simulink model "task9_visu_v23_beide_modelle"  (R2023b)
settings: Solver=VariableStepAuto  StartTime=0.0  StopTime=3  RelTol=1e-3
values from neighbouring files (symbols this model uses):
  tInterval = [0 5]    [task7b.m]    (also in task7b2.m; task8b_setup.m = [0 10]; task9_visu.m = [0 10]; task9b_setup.m = [0 10])
undefined symbols (not defined in the file or in its folder): eul2tform, trvec2tform
libraries: robotcorelib x6, robotmaniplib x4
settings Model: Creator=laith  LastModifiedBy=Nico
settings RTWCC: GPUComputeCapability=5.0

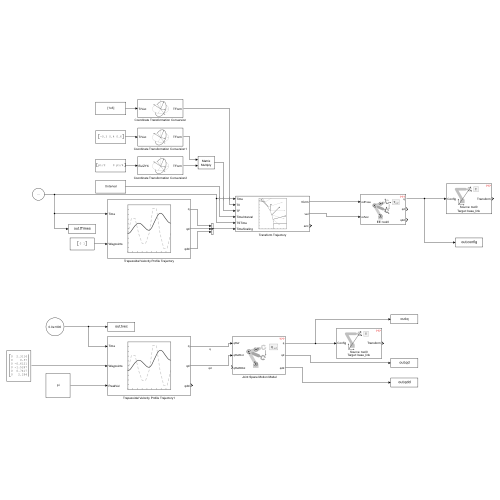
[thumbnail: Simulink's stored preview of the top-level diagram]
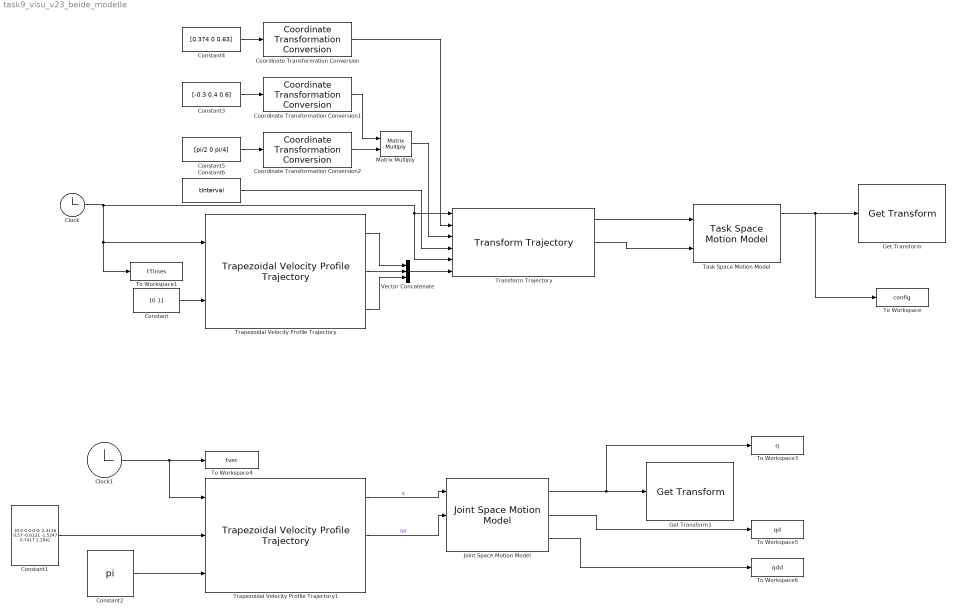
== system task9_visu_v23_beide_modelle ==
  " Joint Space Motion Model" : robotmaniplib/Joint Space Motion Model  RigidBodyTree=robotRBT  MotionType=PD Control  ProportionalGain=200  DerivativeGain=50  ErrorDynamicsSpecification=Damping Ratio / Natural Frequency  DampingRatio=1  NaturalFrequency=10  SettlingTime=0.59  Overshoot=0  ShowExternalForcePort=off  InitConfig=[0 0 0 0 0 0]  InitJointVel=0  SimulateUsing=Interpreted execution
  Clock : Clock
      settings: Decimation=100
  Clock1 : Clock
      settings: Decimation=100
  Constant : Constant  Value=[0 1]  VectorParams1D=off
  Constant1 : Constant  Value="[0 0 0 0 0 0;  2.3116  0.57  -0.6121   -1.5247 0.7417    2.294]'"
  Constant2 : Constant  Value=pi
  Constant3 : Constant  Value=[-0.3 0.4 0.6]
  Constant4 : Constant  Value=[0.374 0 0.63]
  Constant5 : Constant  Value=[pi/2 0 pi/4]
  Constant6 : Constant  Value=tInterval
  Coordinate Transformation Conversion : robotcorelib/Coordinate Transformation Conversion  InputRepresentation=Translation Vector  InputEulerSequence=ZYX  ShowTrVecInputPort=on  OutputRepresentation=Homogeneous Transformation  OutputEulerSequence=ZYX  ShowTrVecOutputPort=on  SimulateUsing=Interpreted execution
  Coordinate Transformation Conversion1 : robotcorelib/Coordinate Transformation Conversion  InputRepresentation=Translation Vector  InputEulerSequence=ZYX  ShowTrVecInputPort=on  OutputRepresentation=Homogeneous Transformation  OutputEulerSequence=ZYX  ShowTrVecOutputPort=off  SimulateUsing=Interpreted execution
  Coordinate Transformation Conversion2 : robotcorelib/Coordinate Transformation Conversion  InputRepresentation=Euler Angles  InputEulerSequence=ZYX  ShowTrVecInputPort=off  OutputRepresentation=Homogeneous Transformation  OutputEulerSequence=ZYX  ShowTrVecOutputPort=on  SimulateUsing=Interpreted execution
  Get Transform : robotmaniplib/Get Transform  RigidBodyTree=robotRBT  SourceBody=tool0  TargetBody=base_link  SimulateUsing=Interpreted execution
  Get Transform1 : robotmaniplib/Get Transform  RigidBodyTree=robotRBT  SourceBody=tool0  TargetBody=base_link  SimulateUsing=Interpreted execution
  Matrix Multiply : Product  Multiplication=Matrix(*)
  Task Space Motion Model : robotmaniplib/Task Space Motion Model  RigidBodyTree=robotRBT  EndEffector=tool0  ProportionalGain=500*eye(6)  DerivativeGain=100*eye(6)  JointDamping=1  ShowExternalForcePort=off  InitConfig=[0 0 0 0 0 0]  InitJointVel=0  SimulateUsing=Interpreted execution
  To Workspace : ToWorkspace  VariableName=config  SampleTime=-1
  To Workspace1 : ToWorkspace  VariableName=tTimes  SampleTime=-1
  To Workspace3 : ToWorkspace  VariableName=q  SampleTime=-1
      settings: Save2DSignal=2-D array (concatenate along first dimension)
  To Workspace4 : ToWorkspace  VariableName=tvec  SampleTime=-1
  To Workspace5 : ToWorkspace  VariableName=qd  SampleTime=-1
      settings: Save2DSignal=2-D array (concatenate along first dimension)
  To Workspace6 : ToWorkspace  VariableName=qdd  SampleTime=-1
      settings: Save2DSignal=2-D array (concatenate along first dimension)
  Transform Trajectory : robotcorelib/Transform Trajectory  WaypointSource=External  T0=trvec2tform( [ 1, 10, -1 ] )  TF=eul2tform( [ 0, pi, pi / 2 ] )  TimeInterval=[ 2, 3 ]  CustomTimeScaling=on  ParameterSource=External  TSTime=2:0.1:3  TimeScaling=[ 0:0.1:1; ones( 1, 11 ); zeros( 1, 11 ) ]  SimulateUsing=Interpreted execution
      settings: LibrarySourceBlock=robotutilslib/Transform Trajectory
  Trapezoidal Velocity Profile Trajectory : robotcorelib/Trapezoidal Velocity Profile Trajectory  WaypointSource=External  Waypoints=[ 0, -0.5, -1; 0, 0.5, 1 ]  NumParams=0  Parameter1=End Time  Parameter2=End Time  ParameterSource=External  PeakVelocity=[ 2; 2 ]  Acceleration=[ 1; 2 ]  EndTime=[ 1; 1 ]  AccelTime=[ 1; 2 ]  SimulateUsing=Code generation
  Trapezoidal Velocity Profile Trajectory1 : robotcorelib/Trapezoidal Velocity Profile Trajectory  WaypointSource=External  Waypoints=[ 0, -0.5, -1; 0, 0.5, 1 ]  NumParams=1  Parameter1=Peak Velocity  Parameter2=Acceleration  ParameterSource=External  PeakVelocity=[ 2; 2 ]  Acceleration=[ 1; 2 ]  EndTime=[ 1; 1 ]  AccelTime=[ 1; 2 ]  SimulateUsing=Interpreted execution
  Vector Concatenate : Concatenate  NumInputs=3  Mode=Multidimensional array
  wires:
  Constant5/1 -> Coordinate Transformation Conversion2/1
  Task Space Motion Model/1 -> To Workspace/1, Get Transform/1
  Transform Trajectory/2 -> Task Space Motion Model/2
  Vector Concatenate/1 -> Transform Trajectory/6
  Constant3/1 -> Coordinate Transformation Conversion1/1
  Coordinate Transformation Conversion/1 -> Transform Trajectory/2
  Trapezoidal Velocity Profile Trajectory/3 -> Vector Concatenate/3
  Trapezoidal Velocity Profile Trajectory/1 -> Vector Concatenate/1
  Constant/1 -> Trapezoidal Velocity Profile Trajectory/2
  Coordinate Transformation Conversion1/1 -> Matrix Multiply/1
  Coordinate Transformation Conversion2/1 -> Matrix Multiply/2
  Matrix Multiply/1 -> Transform Trajectory/3
  Constant4/1 -> Coordinate Transformation Conversion/1
  Trapezoidal Velocity Profile Trajectory/2 -> Vector Concatenate/2
  Clock/1 -> To Workspace1/1, Trapezoidal Velocity Profile Trajectory/1, Transform Trajectory/1, Transform Trajectory/5
  Constant6/1 -> Transform Trajectory/4
  Transform Trajectory/1 -> Task Space Motion Model/1
  Trapezoidal Velocity Profile Trajectory1/2 -> " Joint Space Motion Model"/2  "qd"
  " Joint Space Motion Model"/1 -> To Workspace3/1, Get Transform1/1
  Clock1/1 -> Trapezoidal Velocity Profile Trajectory1/1, To Workspace4/1
  Constant1/1 -> Trapezoidal Velocity Profile Trajectory1/2
  " Joint Space Motion Model"/3 -> To Workspace6/1
  Constant2/1 -> Trapezoidal Velocity Profile Trajectory1/3
  Trapezoidal Velocity Profile Trajectory1/1 -> " Joint Space Motion Model"/1  "q"
  " Joint Space Motion Model"/2 -> To Workspace5/1
